simulink model "batt_model"  (R2022b)
settings: Solver=VariableStepAuto  StartTime=0.0  StopTime=10.0  RelTol=1e-3
values from neighbouring files (symbols this model uses):
  C1_ECM = 1e-6    (= 1e-06)    [load_ECM_params.m]
  C2_ECM = 1e-6    (= 1e-06)    [load_ECM_params.m]
  DT = 5    [load_ECM_params.m]    (also in load_params.m)
  R0_ECM = 0.02    [load_ECM_params.m]
  R1_ECM = 0.03    [load_ECM_params.m]
  R2_ECM = 0.03    [load_ECM_params.m]
  V0_ECM = 4.2    [load_ECM_params.m]
undefined symbols (not defined in the file or in its folder): DiscIntNeverNeededParam
settings Model: R0=0.1  V0=3.7  R1=0.1  R2=0.1  C1=0.1  C2=0.1  Creator=adamp  LastModifiedBy=adamp
settings SolverCC: AlgebraicLoopSolver=TrustRegion
settings DebuggingCC: UnconnectedInputMsg=warning  UnconnectedOutputMsg=warning  UnconnectedLineMsg=warning  SFMachineParentedDataDiag=warning
settings ModelReferenceCC: EnableRefExpFcnMdlSchedulingChecks=on

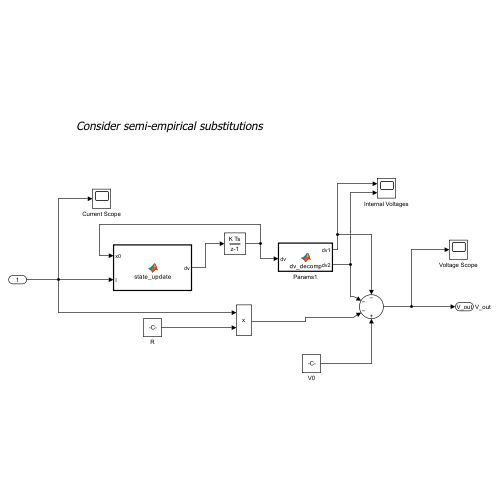
[thumbnail: Simulink's stored preview of the top-level diagram]
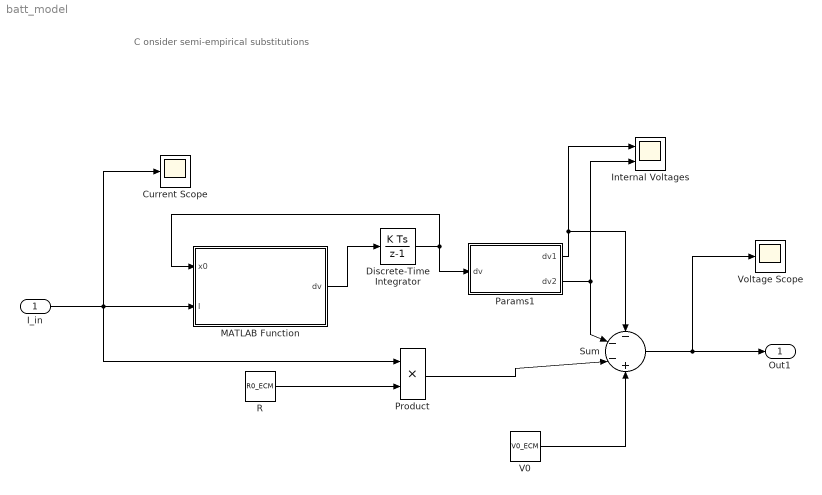
== system batt_model ==
  note: C onsider semi-empirical substitutions
  I_in : Inport
  Current Scope : Scope
  Discrete-Time Integrator : DiscreteIntegrator  InitialCondition=[0 0]  SampleTime=DT  ICPrevOutput=DiscIntNeverNeededParam  ICPrevScaledInput=DiscIntNeverNeededParam
  Internal Voltages : Scope  NumInputPorts=2
  MATLAB Function : MATLAB Function  TreatAsAtomicUnit=on
  Params1 : MATLAB Function  TreatAsAtomicUnit=on
  Product : Product
  R : Constant  Value=R0_ECM
  Sum : Sum  Inputs=---+
  V0 : Constant  Value=V0_ECM
  Voltage Scope : Scope
  Out1 : Outport  SignalName=V_out
  wires:
  MATLAB Function/1(dv) -> Discrete-Time Integrator/1
  Discrete-Time Integrator/1 -> Params1/1(dv), MATLAB Function/1(x0)
  Sum/1 -> Voltage Scope/1, Out1/1
  V0/1 -> Sum/4
  Params1/2(dv2) -> Internal Voltages/2, Sum/2
  Params1/1(dv1) -> Internal Voltages/1, Sum/1
  Product/1 -> Sum/3
  I_in/1 -> Current Scope/1, MATLAB Function/2(I), Product/1
  R/1 -> Product/2

== matlab function batt_model/MATLAB Function ==
  data: x0 input; dv output; I input; R1_ECM parameter; R2_ECM parameter; C1_ECM parameter; C2_ECM parameter
function dv = state_update(x0, I, R1_ECM, R2_ECM, C1_ECM, C2_ECM)
% x = [v1 v2]
R1 = R1_ECM;
R2 = R2_ECM;
C1 = C1_ECM;
C2 = C2_ECM;

dv1 = -x0(1)/(R1*C1) + I/C1;
dv2 = -x0(2)/(R2*C2) + I/C2;
dv = [dv1 dv2];
end

== matlab function batt_model/Params1 ==
  data: dv input; dv1 output; dv2 output
function [dv1, dv2] = dv_decomp(dv)

dv1 = dv(1);
dv2 = dv(2);
end
